simulink model "freebody_simulation"  (R2018a)
settings: Solver=VariableStepAuto  StartTime=0.0  StopTime=20  RelTol=1e-3
libraries: vrlib x1
settings Model: Creator=lamy  LastModifiedBy=lamy

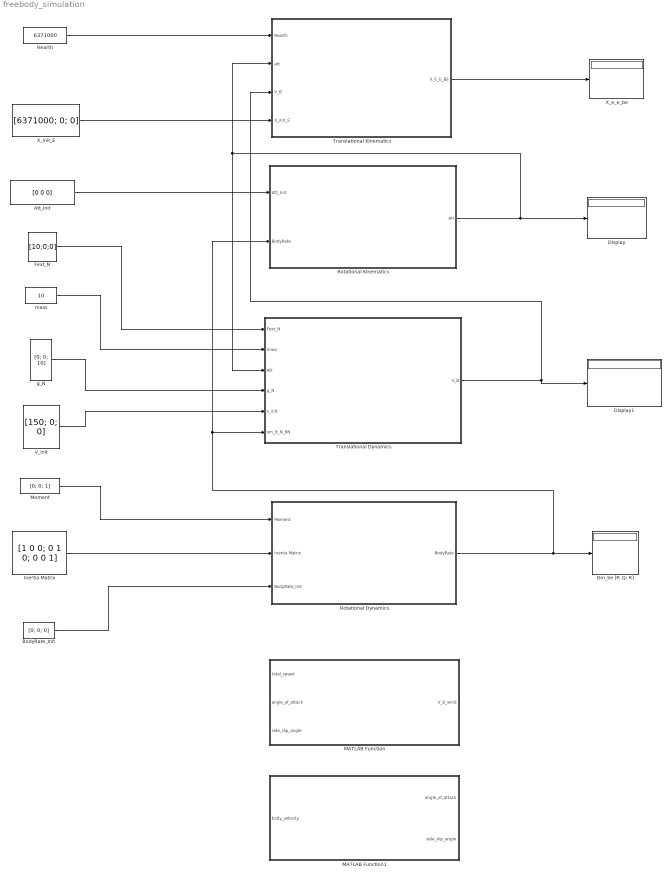
== system freebody_simulation ==
  Att_Init : Constant  Value=[0 0 0]
  BodyRate_Init : Constant  Value=[0; 0; 0]
  Display : Display
  Display1 : Display
  Fext_N : Constant  Value=[10;0;0]  VectorParams1D=off
  Inertia Matrix : Constant  Value=[1 0 0; 0 1 0; 0 0 1]
  MATLAB Function : MATLAB Function  TreatAsAtomicUnit=on
  MATLAB Function1 : MATLAB Function  TreatAsAtomicUnit=on
  Moment : Constant  Value=[0; 0; 1]
  Om_be [P; Q; R] : Display
  Rearth : Constant  Value=6371000
  Rotational Dynamics : Subsystem
  Rotational Kinematics : Subsystem
  Translational Dynamics : Subsystem
  Translational Kinematics : Subsystem
  V_Init : Constant  Value=[150; 0; 0]  VectorParams1D=off
  X_e_e_be : Display
  X_init_E : Constant  Value=[6371000; 0; 0]
  g_N : Constant  Value=[0; 0; 10]  VectorParams1D=off
  mass : Constant  Value=10  VectorParams1D=off
  wires:
  V_Init/1 -> Translational Dynamics/5(v_init)
  g_N/1 -> Translational Dynamics/4(g_N)
  Fext_N/1 -> Translational Dynamics/1(Fext_N)
  mass/1 -> Translational Dynamics/2(mass)
  Rotational Kinematics/1(Att) -> Display/1, Translational Dynamics/3(Att), Translational Kinematics/2(att)
  Moment/1 -> Rotational Dynamics/1(Moment)
  Inertia Matrix/1 -> Rotational Dynamics/2(Inertia Matrix)
  BodyRate_Init/1 -> Rotational Dynamics/3(BodyRate_Init)
  Rearth/1 -> Translational Kinematics/1(Rearth)
  Translational Dynamics/1(V_B) -> Translational Kinematics/3(V_B), Display1/1
  X_init_E/1 -> Translational Kinematics/4(X_init_E)
  Translational Kinematics/1(X_E_E_BE) -> X_e_e_be/1
  Rotational Dynamics/1(BodyRate) -> Om_be [P; Q; R]/1, Translational Dynamics/6(om_B_N_BN), Rotational Kinematics/2(BodyRate)
  Att_Init/1 -> Rotational Kinematics/1(Att_Init)

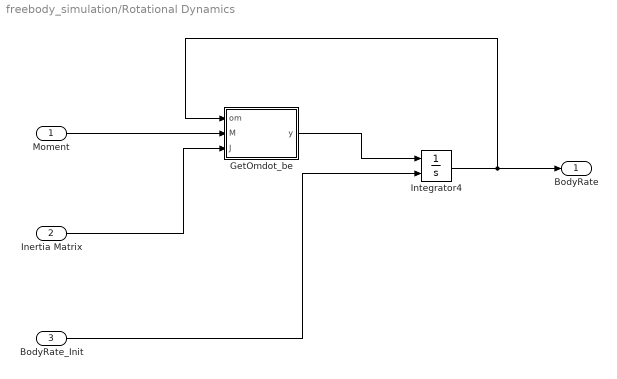
== system freebody_simulation/Rotational Dynamics ==
  Moment : Inport
  Inertia Matrix : Inport  Port=2
  BodyRate_Init : Inport  Port=3
  GetOmdot_be : MATLAB Function  TreatAsAtomicUnit=on
  Integrator4 : Integrator  InitialConditionSource=external
  BodyRate : Outport
  wires:
  GetOmdot_be/1(y) -> Integrator4/1
  Integrator4/1 -> BodyRate/1, GetOmdot_be/1(om)
  BodyRate_Init/1 -> Integrator4/2
  Inertia Matrix/1 -> GetOmdot_be/3(J)
  Moment/1 -> GetOmdot_be/2(M)

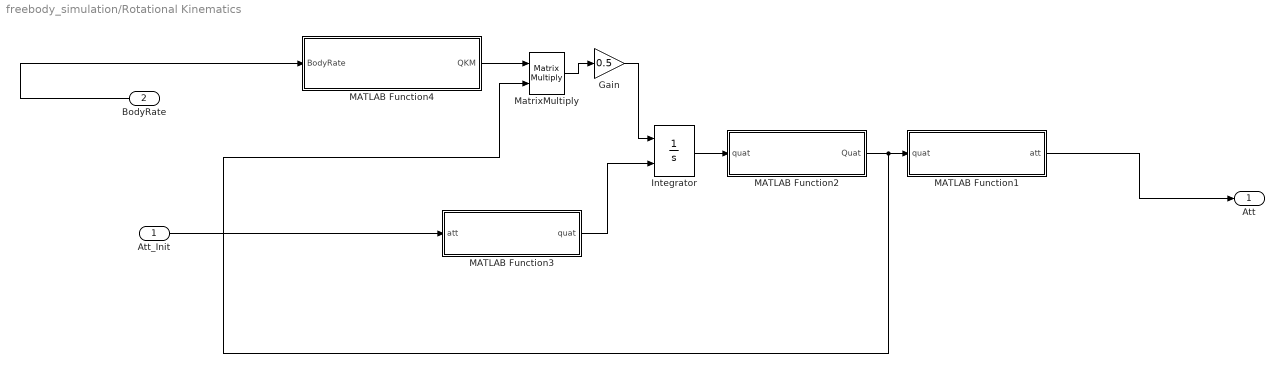
== system freebody_simulation/Rotational Kinematics ==
  Att_Init : Inport
  BodyRate : Inport  Port=2
  Gain : Gain  Gain=0.5
  Integrator : Integrator  InitialConditionSource=external
  MATLAB Function1 : MATLAB Function  TreatAsAtomicUnit=on
  MATLAB Function2 : MATLAB Function  TreatAsAtomicUnit=on
  MATLAB Function3 : MATLAB Function  TreatAsAtomicUnit=on
  MATLAB Function4 : MATLAB Function  TreatAsAtomicUnit=on
  MatrixMultiply : Product  Multiplication=Matrix(*)
  Att : Outport
  wires:
  Att_Init/1 -> MATLAB Function3/1(att)
  Integrator/1 -> MATLAB Function2/1(quat)
  MATLAB Function3/1(quat) -> Integrator/2
  Gain/1 -> Integrator/1
  MATLAB Function4/1(QKM) -> MatrixMultiply/1
  MatrixMultiply/1 -> Gain/1
  MATLAB Function2/1(Quat) -> MatrixMultiply/2, MATLAB Function1/1(quat)
  BodyRate/1 -> MATLAB Function4/1(BodyRate)
  MATLAB Function1/1(att) -> Att/1

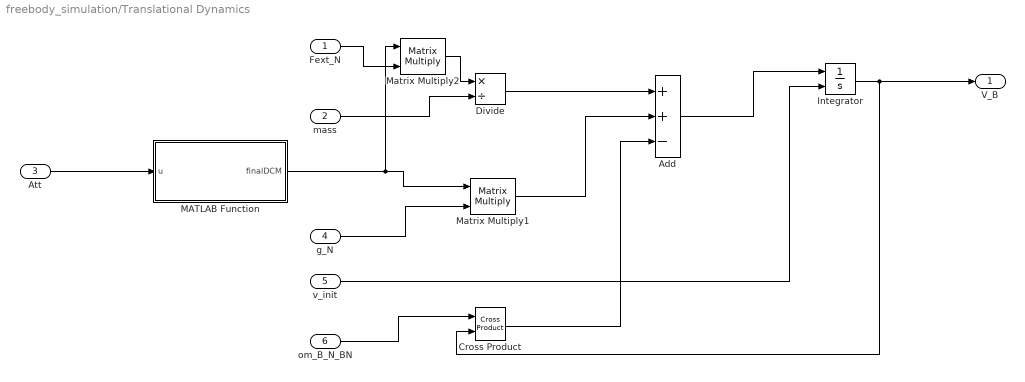
== system freebody_simulation/Translational Dynamics ==
  Fext_N : Inport
  mass : Inport  Port=2
  Att : Inport  Port=3
  g_N : Inport  Port=4
  v_init : Inport  Port=5
  om_B_N_BN : Inport  Port=6
  Add : Sum  Inputs=++-
  Cross Product : vrlib/Utilities/Cross Product
      settings: SourceProductBaseCode=VR
  Divide : Product  Inputs=*/
  Integrator : Integrator  InitialConditionSource=external
  MATLAB Function : MATLAB Function  TreatAsAtomicUnit=on
  Matrix Multiply1 : Product  Multiplication=Matrix(*)
  Matrix Multiply2 : Product  Multiplication=Matrix(*)
  V_B : Outport
  wires:
  Matrix Multiply1/1 -> Add/2
  Cross Product/1 -> Add/3
  om_B_N_BN/1 -> Cross Product/1
  Divide/1 -> Add/1
  Att/1 -> MATLAB Function/1(u)
  Matrix Multiply2/1 -> Divide/1
  Integrator/1 -> V_B/1, Cross Product/2
  mass/1 -> Divide/2
  Add/1 -> Integrator/1
  g_N/1 -> Matrix Multiply1/2
  v_init/1 -> Integrator/2
  Fext_N/1 -> Matrix Multiply2/2
  MATLAB Function/1(finalDCM) -> Matrix Multiply2/1, Matrix Multiply1/1

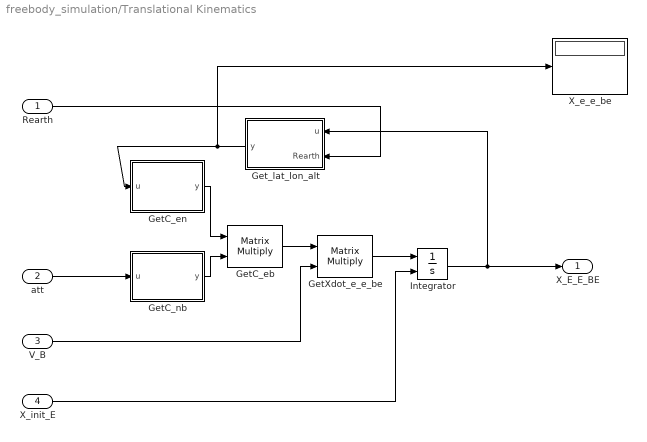
== system freebody_simulation/Translational Kinematics ==
  Rearth : Inport
  att : Inport  Port=2
  V_B : Inport  Port=3
  X_init_E : Inport  Port=4
  GetC_eb : Product  Multiplication=Matrix(*)
  GetC_en : MATLAB Function  TreatAsAtomicUnit=on
  GetC_nb : MATLAB Function  TreatAsAtomicUnit=on
  GetXdot_e_e_be : Product  Multiplication=Matrix(*)
  "Get_lat_lon_alt " : MATLAB Function  TreatAsAtomicUnit=on
  Integrator : Integrator  InitialConditionSource=external
  X_e_e_be : Display
  X_E_E_BE : Outport
  wires:
  GetC_nb/1(y) -> GetC_eb/2
  GetC_en/1(y) -> GetC_eb/1
  Integrator/1 -> X_E_E_BE/1, "Get_lat_lon_alt "/1(u)
  Rearth/1 -> "Get_lat_lon_alt "/2(Rearth)
  GetXdot_e_e_be/1 -> Integrator/1
  "Get_lat_lon_alt "/1(y) -> X_e_e_be/1, GetC_en/1(u)
  att/1 -> GetC_nb/1(u)
  V_B/1 -> GetXdot_e_e_be/2
  GetC_eb/1 -> GetXdot_e_e_be/1
  X_init_E/1 -> Integrator/2

== matlab function freebody_simulation/Rotational Kinematics/MATLAB Function1 ==
  data: quat input; att output
function att = quat2att(quat)
yaw = atan2(2*(quat(1)*quat(4) + quat(2)*quat(3)), 1-2*(quat(3)^2 + quat(4)^2));
pitch = asin(2*(quat(1)*quat(3) - quat(2)*quat(4)));
roll = atan2(2*(quat(1)*quat(2) + quat(3)*quat(4)), 1-2*(quat(2)^2 + quat(3)^2));
att = [roll; pitch; yaw];

== matlab function freebody_simulation/Rotational Kinematics/MATLAB Function4 ==
  data: BodyRate input; QKM output
function QKM = RotKin(BodyRate)
p=BodyRate(1);
q=BodyRate(2);
r=BodyRate(3);
QKM=[ 0,-p,-q,-r;
p, 0, r,-q;
q,-r, 0, p;
r, q,-p, 0];
%q = 0.5*(QKM*quat);

== matlab function freebody_simulation/Rotational Kinematics/MATLAB Function2 ==
  data: quat input; Quat output
function Quat = quat_normalize(quat)
norm = dot(quat,quat);
Quat = quat/norm;

== matlab function freebody_simulation/Rotational Kinematics/MATLAB Function3 ==
  data: att input; quat output
function quat = att2quat(att)
quat = [0;0;0;0];
quat(1) = cos(att(1)/2)*cos(att(2)/2)*cos(att(3)/2) + sin(att(1)/2)*sin(att(2)/2)*sin(att(3)/2);
quat(2) = sin(att(1)/2)*cos(att(2)/2)*cos(att(3)/2) - cos(att(1)/2)*sin(att(2)/2)*sin(att(3)/2);
quat(3) = cos(att(1)/2)*sin(att(2)/2)*cos(att(3)/2) + sin(att(1)/2)*cos(att(2)/2)*sin(att(3)/2);
quat(4) = cos(att(1)/2)*cos(att(2)/2)*sin(att(3)/2) - sin(att(1)/2)*sin(att(2)/2)*cos(att(3)/2);

== matlab function freebody_simulation/Translational Dynamics/MATLAB Function ==
  data: u input; finalDCM output
function finalDCM = att2dcm(u)
yawDCM = [ cos(u(3)) sin(u(3)) 0 ;
-sin(u(3)) cos(u(3)) 0 ;
0 0 1 ];
pitchDCM = [ cos(u(2)) 0 -sin(u(2));
0 1 0 ;
sin(u(2)) 0 cos(u(2)) ];
rollDCM = [ 1 0 0 ;
0 cos(u(1)) sin(u(1));
0 -sin(u(1)) cos(u(1)) ];
finalDCM = rollDCM * pitchDCM * yawDCM;

== matlab function freebody_simulation/Translational Kinematics/GetC_en ==
  data: u input; y output
function y = fcn(u)

C_00  = [ 0         0         1        ;
          0         1         0        ;
         -1         0         0        ];
     
C_lon = [ 1         0         0        ;
          0         cos(u(2)) sin(u(2));
          0        -sin(u(2)) cos(u(2))];
               
C_lat = [ cos(u(1)) 0         sin(u(1));
          0         1         0        ;
         -sin(u(1)) 0         cos(u(1))];
         
   
C_ne = C_lat * C_lon * C_00;
y = C_ne';

== matlab function freebody_simulation/Translational Kinematics/Get_lat_lon_alt  ==
  data: u input; y output; Rearth input
function y = fcn(u, Rearth)

L = sqrt(u(1)^2+u(2)^2+u(3)^2);

lat = asin(u(3)/L);
lon = atan2(u(2),u(1));
alt = L - Rearth;

y = [lat; lon; alt];

== matlab function freebody_simulation/Translational Kinematics/GetC_nb ==
  data: u input; y output
function y = fcn(u)

yawDCM   = [ cos(u(3)) sin(u(3)) 0        ;
            -sin(u(3)) cos(u(3)) 0        ;
             0         0         1        ];
         
pitchDCM = [ cos(u(2)) 0        -sin(u(2));
             0         1         0        ;
             sin(u(2)) 0         cos(u(2))];
         
rollDCM  = [ 1         0         0        ;
             0         cos(u(1)) sin(u(1));
             0        -sin(u(1)) cos(u(1))];
         
finalDCM = rollDCM * pitchDCM * yawDCM;
y = finalDCM';

== matlab function freebody_simulation/MATLAB Function ==
  data: total_speed input; V_B_wind output; angle_of_attack input; side_slip_angle input
function V_B_wind = Sphere2Rect(total_speed, angle_of_attack, side_slip_angle)
alpha = angle_of_attack;
beta = side_slip_angle;
V_B_wind = [total_speed*cos(alpha)*cos(beta);
    total_speed*sin(beta);
    total_speed*sin(alpha)*cos(beta)];
end

== matlab function freebody_simulation/MATLAB Function1 ==
  data: body_velocity input; angle_of_attack output; side_slip_angle output
function [angle_of_attack, side_slip_angle] = Rect2Sphere(body_velocity)
total_speed = norm(body_velocity);
angle_of_attack = atan2(body_velocity(3),body_velocity(1));
side_slip_angle = asin(body_velocity(2)/total_speed);
end

== matlab function freebody_simulation/Rotational Dynamics/GetOmdot_be ==
  data: om input; M input; y output; J input
function y = fcn(om, M, J)

omCPM = [ 0     -om(3)  om(2);
          om(3)  0     -om(1);
         -om(2)  om(1)  0   ];
     
J_inv = inv(J);     

y = J_inv*(M-omCPM*J*om);
